simulink model "clutch"  (R2020a)
settings: Solver=VariableStepAuto  StartTime=0.0  StopTime=10.0  RelTol=1e-3
values from neighbouring files (symbols this model uses):
  be = 2.0    [clutchdata.sldd]
  bv = 1.0    [clutchdata.sldd]
  Fn = 0.0 1.0 2.0 3.0 4.0 5.0 6.0 7.0 8.0 9.0 10.0 0.0 0.8 1.6 1.6 1.6 1.6 0.8 0.0 0.0 0.0 0.0    [clutchdata.sldd]
  Ie = 1.0    [clutchdata.sldd]
  Iv = 5.0    [clutchdata.sldd]
  muk = 1.0    [clutchdata.sldd]
  mus = 1.5    [clutchdata.sldd]
  R = 1.0    [clutchdata.sldd]
  Tin = 1.0 2.0 3.0 4.0 5.0 6.0 7.0 8.0 9.0 10.0 2.0 2.0 2.0 2.0 2.0 0.0 0.0 0.0 0.0 0.0    [clutchdata.sldd]
settings Model: DataDictionary=clutchdata.sldd  Creator=kasutav  LastModifiedBy=kasutav

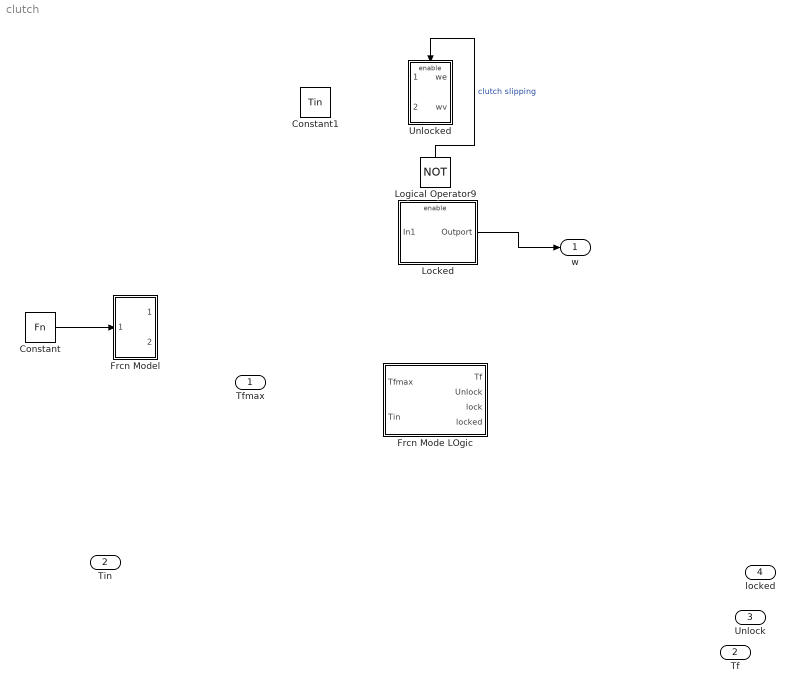
== system clutch ==
  Tfmax : Inport
  Tin : Inport  Port=2
  Constant : Constant  Value=Fn
  Constant1 : Constant  Value=Tin
  Frcn Mode LOgic : Subsystem
  Frcn Model : Subsystem
  Locked : Subsystem
  Logical Operator9 : Logic  Operator=NOT  Inputs=1  IconShape=distinctive  OutDataTypeStr=boolean
  Unlocked : Subsystem
  w : Outport  InitialOutput=0  VectorParamsAs1DForOutWhenUnconnected=off
  Tf : Outport  Port=2
  Unlock : Outport  Port=3
  locked : Outport  Port=4
  wires:
  Constant/1 -> Frcn Model/1(In1)
  Logical Operator9/1 -> Unlocked/Enable  "clutch slipping"
  Locked/1(Outport) -> w/1
  ? -> Locked/Enable, Logical Operator9/1

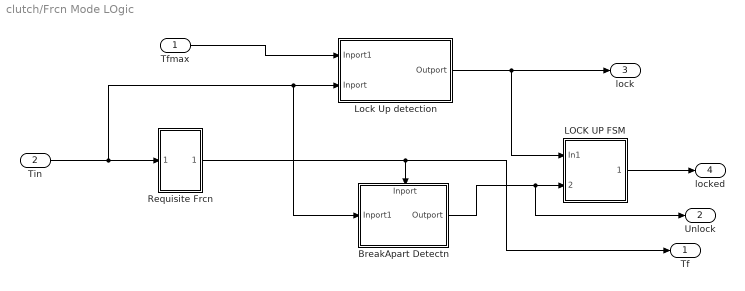
== system clutch/Frcn Mode LOgic ==
  Tfmax : Inport
  Tin : Inport  Port=2
  BreakApart Detectn : Subsystem
      settings: PortSchema="{\"entries\":[{\"content\":{\"sides\":[{\"content\":{\"connectorIds\":[\"In1\"]},\"type\":\"ConnectorPlacement.EquallySpacedRectSide\",\"uuid\":\"50144896-eb41-4f74-af22-fc812245d00a\"},{\"content\":{\"connectorIds\":[\"Out1\"],\"side\":\"RIGHT\"},\"type\":\"ConnectorPlacement.EquallySpacedRectSide\",\"uuid\":\"ec3dc007-03cd-4adb-b7fa-a729d1427153\"},{\"content\":{\"connectorIds\":[\"In2\"],\"side\":\"TOP\"},\"type\":\"ConnectorPlacement.EquallySpacedRectSide\",\"uuid\":\"c40019fe-b816-45bb-9f9d-8caa45d0da79\"}]},\"type\":\"ConnectorPlacement.EquallySpacedConnector\",\"uuid\":\"b0a29feb-6072-48a7-8566-24c544adbab5\"}],\"packageUris\":[\"http://schema.mathworks.com/mf0/Connector/19700101\"],\"version\":\"1.0\"}"
  LOCK UP FSM : Subsystem
  Lock Up detection : Subsystem
  Requisite Frcn : Subsystem
  Tf : Outport
  Unlock : Outport  Port=2
  lock : Outport  Port=3
  locked : Outport  Port=4
  wires:
  Lock Up detection/1(Outport) -> lock/1, LOCK UP FSM/1(In1)
  Requisite Frcn/1(Outport) -> Tf/1, BreakApart Detectn/2(Inport)
  Tfmax/1 -> Lock Up detection/1(Inport1)
  Tin/1 -> Requisite Frcn/1(Inport), BreakApart Detectn/1(Inport1), Lock Up detection/2(Inport)
  LOCK UP FSM/1(locked) -> locked/1
  BreakApart Detectn/1(Outport) -> Unlock/1, LOCK UP FSM/2(Outport)

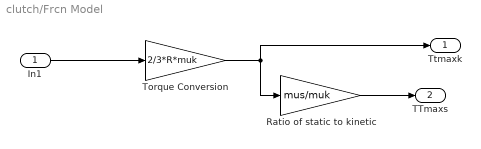
== system clutch/Frcn Model ==
  In1 : Inport
  Ratio of static to kinetic : Gain  Gain=mus/muk  SaturateOnIntegerOverflow=on  OutDataTypeStr=Inherit: Same as input  ParamDataTypeStr=Inherit: Same as input
  Torque Conversion : Gain  Gain=2/3*R*muk  SaturateOnIntegerOverflow=on  OutDataTypeStr=Inherit: Same as input  ParamDataTypeStr=Inherit: Same as input
  Ttmaxk : Outport
  TTmaxs : Outport  Port=2
  wires:
  Ratio of static to kinetic/1 -> TTmaxs/1
  In1/1 -> Torque Conversion/1
  Torque Conversion/1 -> Ttmaxk/1, Ratio of static to kinetic/1

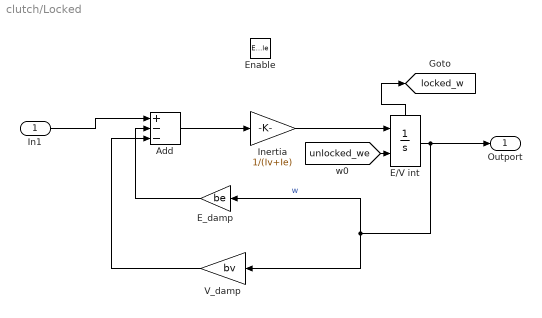
== system clutch/Locked ==
  In1 : Inport
  Enable : EnablePort  StatesWhenEnabling=reset
  " E/V int" : Integrator  InitialConditionSource=external  ShowStatePort=on
  Add : Sum  Inputs=+--
  E_damp : Gain  Gain=be  SaturateOnIntegerOverflow=on  OutDataTypeStr=Inherit: Same as input  ParamDataTypeStr=Inherit: Same as input
  Inertia : Gain  Gain=1/(Iv+Ie)  SaturateOnIntegerOverflow=on  OutDataTypeStr=Inherit: Same as input  ParamDataTypeStr=Inherit: Same as input
  V_damp : Gain  Gain=bv  SaturateOnIntegerOverflow=on  OutDataTypeStr=Inherit: Same as input  ParamDataTypeStr=Inherit: Same as input
  Outport : Outport
  tag scope: locked_w=global
  wires:
  Add/1 -> Inertia/1
  In1/1 -> Add/1
  Inertia/1 -> " E/V int"/1
  [unlocked_we] -> " E/V int"/2
  " E/V int"/State -> [locked_w]
  " E/V int"/1 -> Outport/1, E_damp/1, V_damp/1  "w"
  E_damp/1 -> Add/2
  V_damp/1 -> Add/3

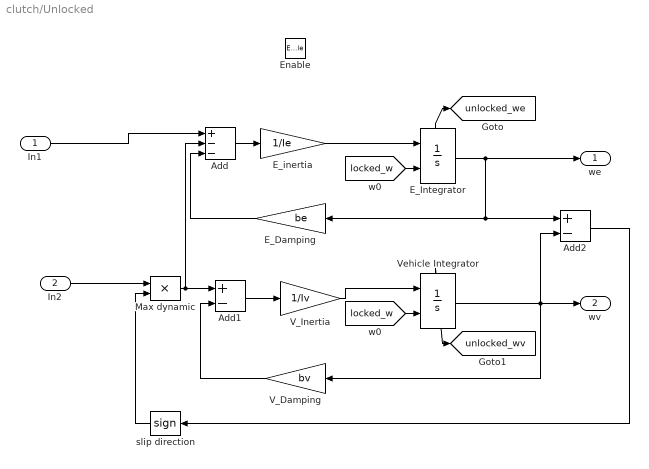
== system clutch/Unlocked ==
  In1 : Inport
  In2 : Inport  Port=2
  Enable : EnablePort  StatesWhenEnabling=reset
  Add : Sum  Inputs=+--
  Add1 : Sum  Inputs=+-
  Add2 : Sum  Inputs=+-
  E_Damping : Gain  Gain=be  SaturateOnIntegerOverflow=on  OutDataTypeStr=Inherit: Same as input  ParamDataTypeStr=Inherit: Same as input
  E_Integrator : Integrator  InitialConditionSource=external  ShowStatePort=on
  E_inertia : Gain  Gain=1/Ie  SaturateOnIntegerOverflow=on  OutDataTypeStr=Inherit: Same as input  ParamDataTypeStr=Inherit: Same as input
  "Max dynamic " : Product  InputSameDT=on  RndMeth=Zero  SaturateOnIntegerOverflow=on  OutDataTypeStr=Inherit: Same as first input
  V_Damping : Gain  Gain=bv  SaturateOnIntegerOverflow=on  OutDataTypeStr=Inherit: Same as input  ParamDataTypeStr=Inherit: Same as input
  V_Inertia : Gain  Gain=1/Iv  SaturateOnIntegerOverflow=on  OutDataTypeStr=Inherit: Same as input  ParamDataTypeStr=Inherit: Same as input
  Vehicle Integrator : Integrator  InitialConditionSource=external  ShowStatePort=on
  slip direction : Signum
  we : Outport
  wv : Outport  Port=2
  tag scope: unlocked_we=global, unlocked_wv=global
  wires:
  E_Integrator/State -> [unlocked_we]
  slip direction/1 -> "Max dynamic "/2
  E_inertia/1 -> E_Integrator/1
  In2/1 -> "Max dynamic "/1
  Vehicle Integrator/State -> [unlocked_wv]
  [locked_w] -> E_Integrator/2
  V_Inertia/1 -> Vehicle Integrator/1
  Vehicle Integrator/1 -> wv/1, Add2/2, V_Damping/1
  "Max dynamic "/1 -> Add1/1, Add/2
  [locked_w] -> Vehicle Integrator/2
  Add1/1 -> V_Inertia/1
  E_Integrator/1 -> we/1, Add2/1, E_Damping/1
  Add/1 -> E_inertia/1
  In1/1 -> Add/1
  E_Damping/1 -> Add/3
  V_Damping/1 -> Add1/2
  Add2/1 -> slip direction/1

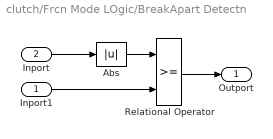
== system clutch/Frcn Mode LOgic/BreakApart Detectn ==
  Inport1 : Inport
  Inport : Inport  Port=2
  Abs : Abs  SaturateOnIntegerOverflow=on
  Relational Operator : RelationalOperator  OutDataTypeStr=boolean  RndMeth=Nearest  InputSameDT=on
  Outport : Outport
  wires:
  Inport/1 -> Abs/1
  Inport1/1 -> Relational Operator/2
  Abs/1 -> Relational Operator/1
  Relational Operator/1 -> Outport/1

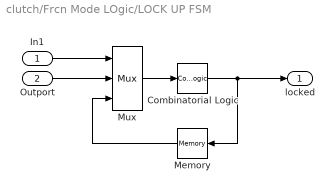
== system clutch/Frcn Mode LOgic/LOCK UP FSM ==
  In1 : Inport
  Outport : Inport  Port=2
  Combinatorial Logic : CombinatorialLogic  TruthTable=[0;1;0;0;1;1;1;0]
  Memory : Memory
  Mux : Mux  Inputs=3
  locked : Outport  InitialOutput=0  VectorParamsAs1DForOutWhenUnconnected=off
  wires:
  In1/1 -> Mux/1
  Outport/1 -> Mux/2
  Mux/1 -> Combinatorial Logic/1
  Memory/1 -> Mux/3
  Combinatorial Logic/1 -> locked/1, Memory/1

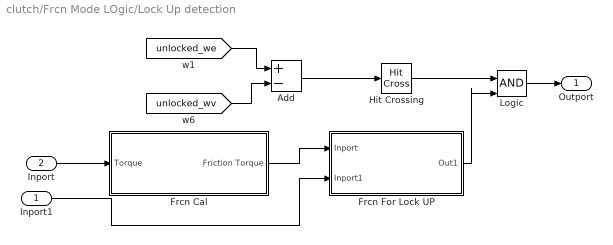
== system clutch/Frcn Mode LOgic/Lock Up detection ==
  Inport1 : Inport
  Inport : Inport  Port=2
  Add : Sum  Inputs=+-
  Frcn Cal : Subsystem
  Frcn For Lock UP : Subsystem
  Hit Crossing : HitCross
  Logic : Logic  IconShape=distinctive  OutDataTypeStr=boolean
  Outport : Outport
  wires:
  Inport1/1 -> Frcn For Lock UP/2(Inport1)
  Inport/1 -> Frcn Cal/1(Torque)
  Hit Crossing/1 -> Logic/1
  Frcn For Lock UP/1(Out1) -> Logic/2
  [unlocked_wv] -> Add/2
  Add/1 -> Hit Crossing/1
  [unlocked_we] -> Add/1
  Frcn Cal/1(Friction Torque) -> Frcn For Lock UP/1(Inport)
  Logic/1 -> Outport/1

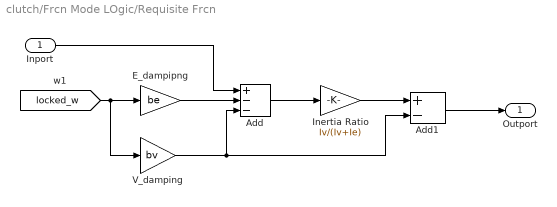
== system clutch/Frcn Mode LOgic/Requisite Frcn ==
  Inport : Inport
  Add : Sum  Inputs=+--
  Add1 : Sum  Inputs=+-
  E_dampipng : Gain  Gain=be  SaturateOnIntegerOverflow=on  OutDataTypeStr=Inherit: Same as input  ParamDataTypeStr=Inherit: Same as input
  Inertia Ratio : Gain  Gain=Iv/(Iv+Ie)  SaturateOnIntegerOverflow=on  OutDataTypeStr=Inherit: Same as input  ParamDataTypeStr=Inherit: Same as input
  V_damping : Gain  Gain=bv  SaturateOnIntegerOverflow=on  OutDataTypeStr=Inherit: Same as input  ParamDataTypeStr=Inherit: Same as input
  Outport : Outport
  wires:
  Add/1 -> Inertia Ratio/1
  [locked_w] -> V_damping/1, E_dampipng/1
  V_damping/1 -> Add1/2, Add/3
  E_dampipng/1 -> Add/2
  Inport/1 -> Add/1
  Inertia Ratio/1 -> Add1/1
  Add1/1 -> Outport/1

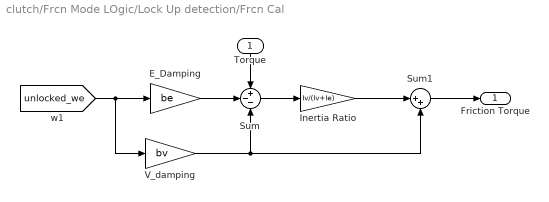
== system clutch/Frcn Mode LOgic/Lock Up detection/Frcn Cal ==
  Torque : Inport
  E_Damping : Gain  Gain=be  SaturateOnIntegerOverflow=on  OutDataTypeStr=Inherit: Same as input  ParamDataTypeStr=Inherit: Same as input
  Inertia Ratio : Gain  Gain=Iv/(Iv+Ie)  SaturateOnIntegerOverflow=on  OutDataTypeStr=Inherit: Same as input  ParamDataTypeStr=Inherit: Same as input
  Sum : Sum  Inputs=+--  InputSameDT=on  SaturateOnIntegerOverflow=on  OutDataTypeStr=Inherit: Same as first input
  Sum1 : Sum  Inputs=|++  InputSameDT=on  SaturateOnIntegerOverflow=on  OutDataTypeStr=Inherit: Same as first input
  V_damping : Gain  Gain=bv  SaturateOnIntegerOverflow=on  OutDataTypeStr=Inherit: Same as input  ParamDataTypeStr=Inherit: Same as input
  Friction Torque : Outport  InitialOutput=0  VectorParamsAs1DForOutWhenUnconnected=off
  wires:
  E_Damping/1 -> Sum/2
  Torque/1 -> Sum/1
  Sum1/1 -> Friction Torque/1
  Sum/1 -> Inertia Ratio/1
  V_damping/1 -> Sum1/2, Sum/3
  [unlocked_we] -> E_Damping/1, V_damping/1
  Inertia Ratio/1 -> Sum1/1

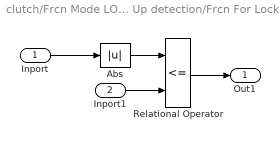
== system clutch/Frcn Mode LOgic/Lock Up detection/Frcn For Lock UP ==
  Inport : Inport
  Inport1 : Inport  Port=2
  Abs : Abs  SaturateOnIntegerOverflow=on
  Relational Operator : RelationalOperator  Operator=<=  OutDataTypeStr=boolean  RndMeth=Nearest  InputSameDT=on
  Out1 : Outport
  wires:
  Abs/1 -> Relational Operator/1
  Inport1/1 -> Relational Operator/2
  Relational Operator/1 -> Out1/1
  Inport/1 -> Abs/1
